simulink model "Gyrostat_Dynamics"  (R2017b)
settings: Solver=VariableStepAuto  StartTime=0.0  StopTime=10.0  RelTol=1e-3
undefined symbols (not defined in the file): Jnom
settings Model: Creator=ayoubia  LastModifiedBy=ayoubia

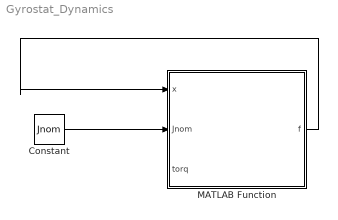
== system Gyrostat_Dynamics ==
  Constant : Constant  Value=Jnom
  MATLAB Function : MATLAB Function  TreatAsAtomicUnit=on
  wires:
  Constant/1 -> MATLAB Function/2(Jnom)
  MATLAB Function/1(f) -> MATLAB Function/1(x)

== matlab function Gyrostat_Dynamics/MATLAB Function ==
  data: x input; f output; Jnom input; torq input
function f=gyrostat(x,Jnom,torq)

f=gyrostat(x,Jnom,torq);
